simulink model "Simulink_PID_controller"  (R2024b)
settings: Solver=FixedStepDiscrete  StartTime=0.0  StopTime=Inf  FixedStep=1e-3  RelTol=1e-3  EnableMultiTasking=on
undefined symbols (not defined in the file): DiscIntNeverNeededParam
libraries: arduinolib x6, simulink x4, arduinosensorlib x2
settings Model: SimulationMode=external  ExtModeTrigDuration=2  Creator=Necus  LastModifiedBy=Rashmika Gunasekera
settings SolverCC: AutoInsertRateTranBlk=on
settings OptimizationCC: DefaultUnderspecifiedDataType=single  EnhancedBackFolding=on  PassReuseOutputArgsAs=Individual arguments  ZeroExternalMemoryAtStartup=off  MaxStackSize=64  OptimizeBlockOrder=speed  DifferentSizesBufferReuse=on  OptimizationCustomize=off  DenormalBehavior=FlushToZero  EfficientTunableParamExpr=on
settings DebuggingCC: ParameterTunabilityLossMsg=error
settings HardwareCC: ProdBitPerInt=16  ProdBitPerPointer=16  ProdBitPerSizeT=16  ProdBitPerPtrDiffT=16  ProdLargestAtomicFloat=None  ProdWordSize=8  ProdHWDeviceType=Atmel->AVR  UseEmbeddedCoderFeatures=off  UseSimulinkCoderFeatures=off
settings SFSimCC: MATLABDynamicMemAlloc=off
settings RTWCC: Description=Embedded Coder  SystemTargetFile=ert.tlc  HardwareBoard=Arduino Mega 2560  TemplateMakefile=ert_default_tmf  Toolchain=Arduino AVR  BuildConfiguration=Faster Runs  GPUComputeCapability=3.5
settings CodeAppCC: ForceParamTrailComments=on  IgnoreCustomStorageClasses=off  OperatorAnnotations=on  SimulinkDataObjDesc=on  SFDataObjDesc=on  InsertBlockDesc=on
settings ERTTargetCC: SupportContinuousTime=on  SupportNonInlinedSFcns=on  SupportVariableSizeSignals=on  ExtMode=on  ExtModeTransport=3  ExtModeStaticAlloc=on  ExtModeAutomaticAllocSize=off  ExtModeStaticAllocSize=2048  ExtModeMexFile=ext_xcp  ExtModeMexArgs=1 8 5625000  ExtModeIntrfLevel=Level2 - Open  InlinedParameterPlacement=Hierarchical  DynamicArrayContainerType=coder::array

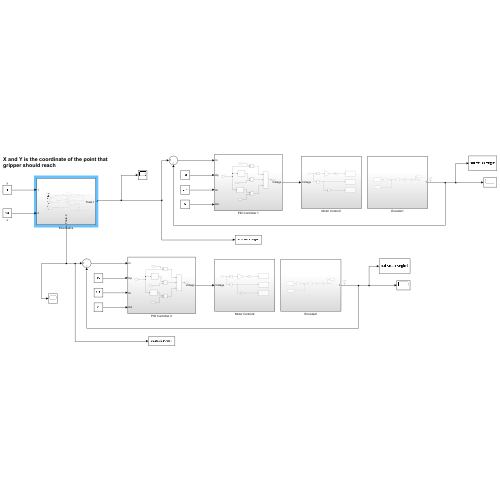
[thumbnail: Simulink's stored preview of the top-level diagram]
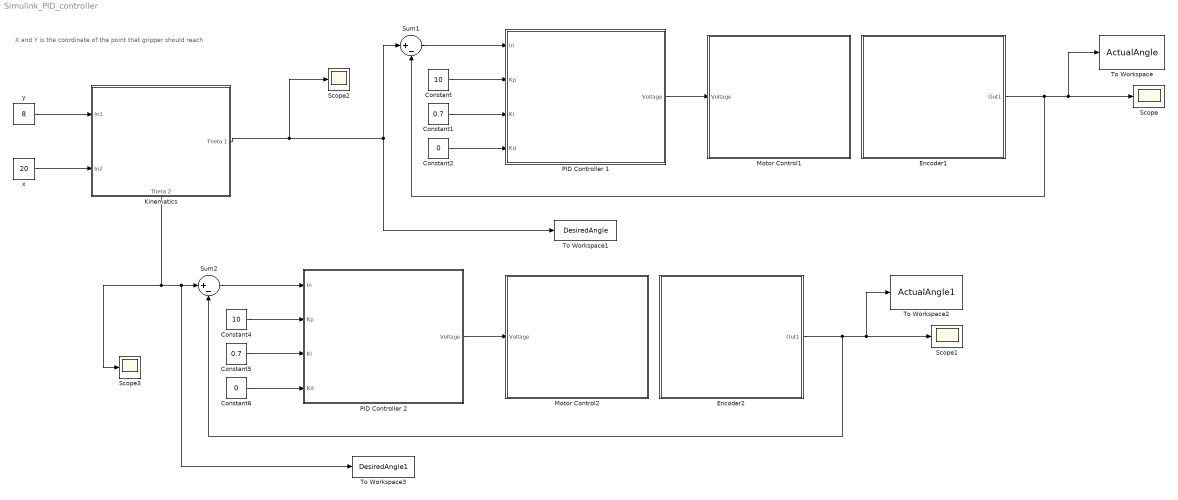
== system Simulink_PID_controller ==
  note: X and Y is the coordinate of the point that gripper should reach
  Constant : Constant  Value=10
  Constant1 : Constant  Value=0.7
  Constant2 : Constant  Value=0
  Constant4 : Constant  Value=10
  Constant5 : Constant  Value=0.7
  Constant6 : Constant  Value=0
  Encoder1 : Subsystem
  Encoder2 : Subsystem
  Kinematics : Subsystem
      settings: PortSchema="{\"entries\":[{\"content\":{\"sides\":[{\"content\":{\"connectorIds\":[\"In1\",\"In2\"]},\"type\":\"ConnectorPlacement.EquallySpacedRectSide\",\"uuid\":\"8a509842-5d2f-4ce8-a55f-cf93434b5f6d\"},{\"content\":{\"connectorIds\":[\"Out1\"],\"side\":\"RIGHT\"},\"type\":\"ConnectorPlacement.EquallySpacedRectSide\",\"uuid\":\"dc9cea0c-3903-48e2-b604-c30f542df696\"},{\"content\":{\"side\":\"TOP\"},\"type\":\"ConnectorPlacement.EquallySpacedRectSide\",\"uuid\":\"6c8ffbb7-f81a-45ff-8455-eba80b841fc4\"},{\"content\":{\"connectorIds\":[\"Out2\"],\"side\":\"BOTTOM\"},\"type\":\"ConnectorPlacement.EquallySpacedRectSide\",\"uuid\":\"0c610225-6bbf-4f4a-ad72-7adf458fb5c5\"}]},\"type\":\"ConnectorPlacement.EquallySpacedConnector\",\"uuid\":\"63fe37e8-0e78-4a01-8657-6f2a85bff4db\"}],\"packageUris\":[\"http://schema.mathworks.com/mf0/Connector/R2020b\"],\"version\":\"1.0\"}"
  Motor Control1 : Subsystem
  Motor Control2 : Subsystem
  PID Controller 1 : Subsystem
  PID Controller 2 : Subsystem
  Scope{,1..3} (4 alike) : Scope
  Sum1 : Sum  Inputs=|+-
  Sum2 : Sum  Inputs=|+-
  To Workspace : ToWorkspace  VariableName=ActualAngle  SaveFormat=Structure With Time  SampleTime=-1
  To Workspace1 : ToWorkspace  VariableName=DesiredAngle  SaveFormat=Structure With Time  SampleTime=-1
  To Workspace2 : ToWorkspace  VariableName=ActualAngle1  SaveFormat=Structure With Time  SampleTime=-1
  To Workspace3 : ToWorkspace  VariableName=DesiredAngle1  SaveFormat=Structure With Time  SampleTime=-1
  x : Constant  Value=20
  y : Constant  Value=8
  wires:
  Constant/1 -> PID Controller 1/2(Kp)
  Constant1/1 -> PID Controller 1/3(Ki)
  Constant2/1 -> PID Controller 1/4(Kd)
  Sum1/1 -> PID Controller 1/1(In)
  Encoder1/1(Out1) -> To Workspace/1, Scope/1, Sum1/2
  PID Controller 1/1(Voltage) -> Motor Control1/1(Voltage)
  Kinematics/2(Theta 2) -> To Workspace3/1, Sum2/1, Scope3/1
  Encoder2/1(Out1) -> To Workspace2/1, Scope1/1, Sum2/2
  Sum2/1 -> PID Controller 2/1(In)
  Constant6/1 -> PID Controller 2/4(Kd)
  Constant4/1 -> PID Controller 2/2(Kp)
  Constant5/1 -> PID Controller 2/3(Ki)
  PID Controller 2/1(Voltage) -> Motor Control2/1(Voltage)
  Kinematics/1(Theta 1) -> Scope2/1, To Workspace1/1, Sum1/1
  y/1 -> Kinematics/1(In1)
  x/1 -> Kinematics/2(In2)

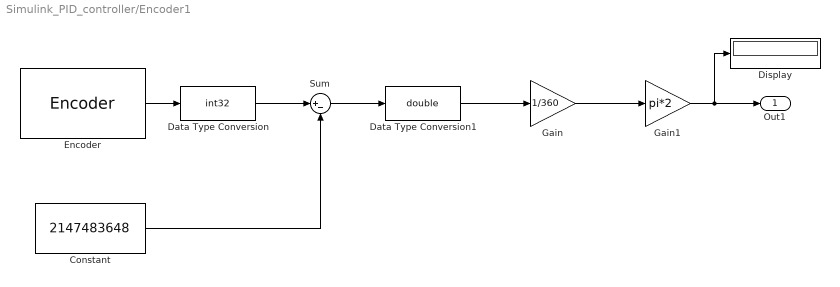
== system Simulink_PID_controller/Encoder1 ==
  Constant : Constant  Value=2147483648  OutDataTypeStr=int32
  Data Type Conversion : DataTypeConversion  OutDataTypeStr=int32  SaturateOnIntegerOverflow=off  RndMeth=Floor
  Data Type Conversion1 : DataTypeConversion  OutDataTypeStr=double  SaturateOnIntegerOverflow=off  RndMeth=Floor
  Display : Display
  Encoder : arduinosensorlib/Encoder  InputA=2  InputB=3  Mode=No reset  SampleTime=-1
      settings: SourceProductName=Sensors
  Gain : Gain  Gain=1/360
  Gain1 : Gain  Gain=pi*2
  Sum : Sum  Inputs=|+-
  Out1 : Outport
  wires:
  Data Type Conversion1/1 -> Gain/1
  Encoder/1 -> Data Type Conversion/1
  Data Type Conversion/1 -> Sum/1
  Sum/1 -> Data Type Conversion1/1
  Constant/1 -> Sum/2
  Gain/1 -> Gain1/1
  Gain1/1 -> Display/1, Out1/1

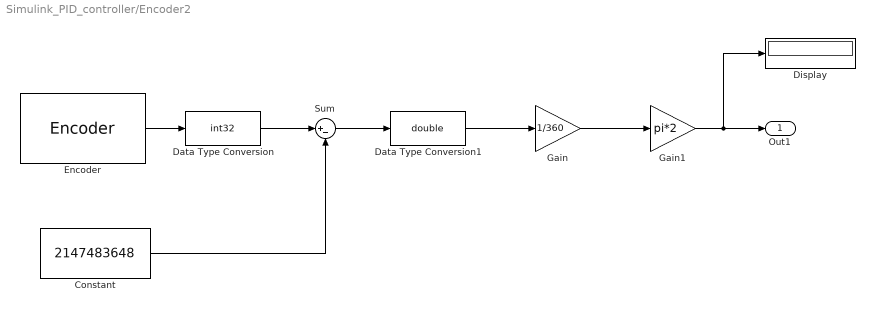
== system Simulink_PID_controller/Encoder2 ==
  Constant : Constant  Value=2147483648  OutDataTypeStr=int32
  Data Type Conversion : DataTypeConversion  OutDataTypeStr=int32  SaturateOnIntegerOverflow=off  RndMeth=Floor
  Data Type Conversion1 : DataTypeConversion  OutDataTypeStr=double  SaturateOnIntegerOverflow=off  RndMeth=Floor
  Display : Display
  Encoder : arduinosensorlib/Encoder  InputA=18  InputB=19  Mode=No reset  SampleTime=-1
      settings: SourceProductName=Sensors
  Gain : Gain  Gain=1/360
  Gain1 : Gain  Gain=pi*2
  Sum : Sum  Inputs=|+-
  Out1 : Outport
  wires:
  Data Type Conversion1/1 -> Gain/1
  Encoder/1 -> Data Type Conversion/1
  Data Type Conversion/1 -> Sum/1
  Sum/1 -> Data Type Conversion1/1
  Constant/1 -> Sum/2
  Gain/1 -> Gain1/1
  Gain1/1 -> Display/1, Out1/1

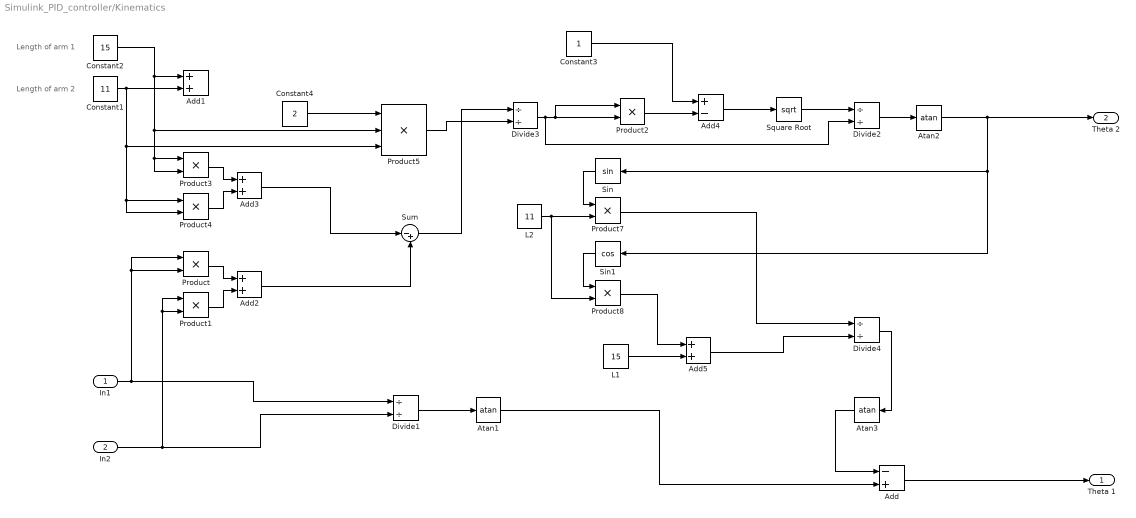
== system Simulink_PID_controller/Kinematics ==
  note: Length of arm 1
  note: Length of arm 2
  In1 : Inport
  In2 : Inport  Port=2
  Add : Sum  Inputs=-+
  Add{1..3,5} (4 alike) : Sum
  Add4 : Sum  Inputs=+-
  Atan1 : Trigonometry  Operator=atan
  Atan2 : Trigonometry  Operator=atan
  Atan3 : Trigonometry  Operator=atan
  Constant1 : Constant  Value=11
  Constant2 : Constant  Value=15
  Constant3 : Constant
  Constant4 : Constant  Value=2
  Divide{1..4} (4 alike) : Product  Inputs=//
  L1 : Constant  Value=15
  L2 : Constant  Value=11
  Product{,1..4,7..8} (7 alike) : Product
  Product5 : Product  Inputs=3
  Sin : Trigonometry
  Sin1 : Trigonometry  Operator=cos
  Square Root : Sqrt
  Sum : Sum  Inputs=|-+
  Theta 1 : Outport
  Theta 2 : Outport  Port=2
  wires:
  In2/1 -> Divide1/2, Product1/2, Product1/1
  In1/1 -> Product/2, Product/1, Divide1/1
  Divide1/1 -> Atan1/1
  Add/1 -> Theta 1/1
  Constant2/1 -> Product3/1, Product3/2, Product5/2, Add1/1
  Constant1/1 -> Product4/1, Product4/2, Product5/3, Add1/2
  Product/1 -> Add2/1
  Product1/1 -> Add2/2
  Product4/1 -> Add3/2
  Product3/1 -> Add3/1
  Add2/1 -> Sum/2
  Add3/1 -> Sum/1
  Sum/1 -> Divide3/1
  Constant4/1 -> Product5/1
  Product5/1 -> Divide3/2
  Atan1/1 -> Add/2
  Divide3/1 -> Product2/2, Product2/1, Divide2/2
  Product2/1 -> Add4/2
  Constant3/1 -> Add4/1
  Add4/1 -> Square Root/1
  Square Root/1 -> Divide2/1
  Divide2/1 -> Atan2/1
  Atan2/1 -> Theta 2/1, Sin1/1, Sin/1
  L2/1 -> Product8/2, Product7/2
  Sin/1 -> Product7/1
  Sin1/1 -> Product8/1
  L1/1 -> Add5/2
  Product8/1 -> Add5/1
  Product7/1 -> Divide4/1
  Add5/1 -> Divide4/2
  Divide4/1 -> Atan3/1
  Atan3/1 -> Add/1

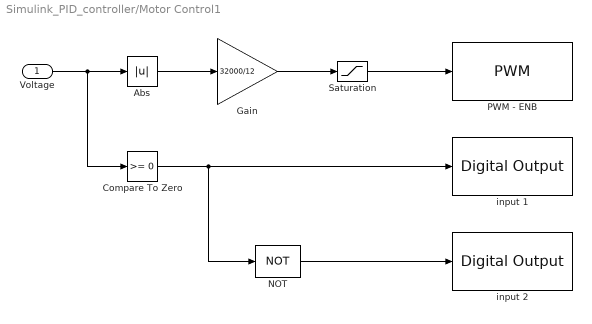
== system Simulink_PID_controller/Motor Control1 ==
  Voltage : Inport
  Abs : Abs  SaturateOnIntegerOverflow=off
  Compare To Zero : simulink/Logic and Bit Operations/Compare To Zero  relop=>=  OutDataTypeStr=boolean
  Gain : Gain  Gain=32000/12
  NOT : Logic  Operator=NOT  IconShape=distinctive  AllPortsSameDT=off  OutDataTypeStr=boolean
  PWM - ENB : arduinolib/PWM  pinNumber=7  frequencyType=Default  desiredFrequency=490.2  achievableFrequency=490.2
      settings: SourceProductName=Common
  Saturation : Saturate  UpperLimit=32000  LowerLimit=0
  "input 1 " : arduinolib/Digital Output  pinNumber=5  Direction=output  blockPlatform=arduino
      settings: SourceProductName=Common
  input 2 : arduinolib/Digital Output  pinNumber=6  Direction=output  blockPlatform=arduino
      settings: SourceProductName=Common
  wires:
  Voltage/1 -> Compare To Zero/1, Abs/1
  Abs/1 -> Gain/1
  Gain/1 -> Saturation/1
  Compare To Zero/1 -> "input 1 "/1, NOT/1
  NOT/1 -> input 2/1
  Saturation/1 -> PWM - ENB/1

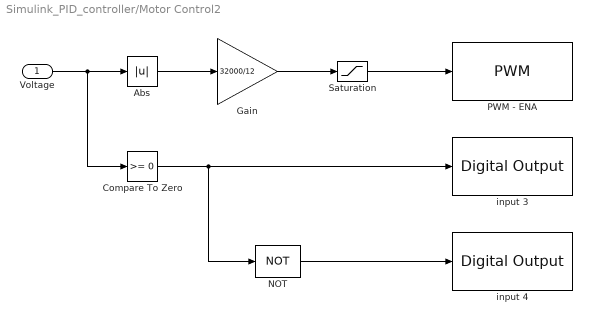
== system Simulink_PID_controller/Motor Control2 ==
  Voltage : Inport
  Abs : Abs  SaturateOnIntegerOverflow=off
  Compare To Zero : simulink/Logic and Bit Operations/Compare To Zero  relop=>=  OutDataTypeStr=boolean
  Gain : Gain  Gain=32000/12
  NOT : Logic  Operator=NOT  IconShape=distinctive  AllPortsSameDT=off  OutDataTypeStr=boolean
  PWM - ENA : arduinolib/PWM  pinNumber=8  frequencyType=Default  desiredFrequency=490.2  achievableFrequency=490.2
      settings: SourceProductName=Common
  Saturation : Saturate  UpperLimit=32000  LowerLimit=0
  "input 3 " : arduinolib/Digital Output  pinNumber=9  Direction=output  blockPlatform=arduino
      settings: SourceProductName=Common
  input 4 : arduinolib/Digital Output  pinNumber=10  Direction=output  blockPlatform=arduino
      settings: SourceProductName=Common
  wires:
  Voltage/1 -> Compare To Zero/1, Abs/1
  Abs/1 -> Gain/1
  Gain/1 -> Saturation/1
  Compare To Zero/1 -> "input 3 "/1, NOT/1
  NOT/1 -> input 4/1
  Saturation/1 -> PWM - ENA/1

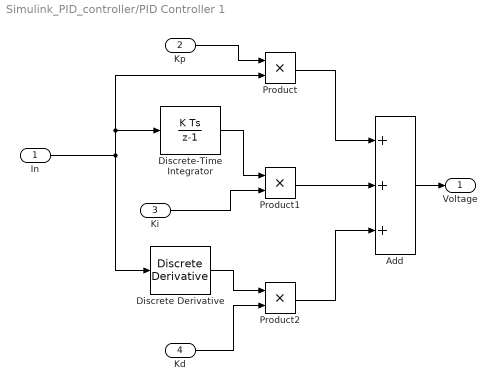
== system Simulink_PID_controller/PID Controller 1 ==
  In : Inport
  Kp : Inport  Port=2
  Ki : Inport  Port=3
  Kd : Inport  Port=4
  Add : Sum  Inputs=+++
  Discrete Derivative : simulink/Discrete/Discrete Derivative  gainval=1.0  ICPrevScaledInput=0.0  OutMin=[]  OutMax=[]  OutDataType=fixdt(1, 16)  OutScaling=2^-10  DoSatur=off
  Discrete-Time Integrator : DiscreteIntegrator  SampleTime=-1  ICPrevOutput=DiscIntNeverNeededParam  ICPrevScaledInput=DiscIntNeverNeededParam
  Product : Product
  Product1 : Product
  Product2 : Product
  Voltage : Outport
  wires:
  Discrete-Time Integrator/1 -> Product1/1
  Product2/1 -> Add/3
  Ki/1 -> Product1/2
  Discrete Derivative/1 -> Product2/1
  In/1 -> Product/2, Discrete-Time Integrator/1, Discrete Derivative/1
  Kd/1 -> Product2/2
  Product/1 -> Add/1
  Product1/1 -> Add/2
  Kp/1 -> Product/1
  Add/1 -> Voltage/1

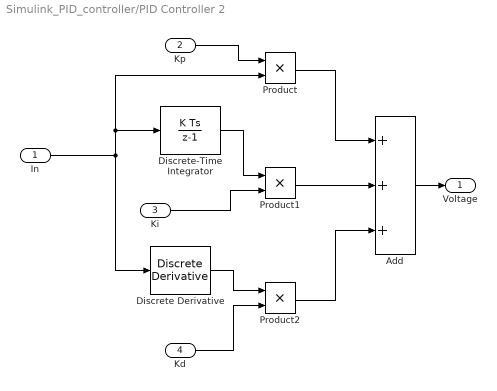
== system Simulink_PID_controller/PID Controller 2 ==
  In : Inport
  Kp : Inport  Port=2
  Ki : Inport  Port=3
  Kd : Inport  Port=4
  Add : Sum  Inputs=+++
  Discrete Derivative : simulink/Discrete/Discrete Derivative  gainval=1.0  ICPrevScaledInput=0.0  OutMin=[]  OutMax=[]  OutDataType=fixdt(1, 16)  OutScaling=2^-10  DoSatur=off
  Discrete-Time Integrator : DiscreteIntegrator  SampleTime=-1  ICPrevOutput=DiscIntNeverNeededParam  ICPrevScaledInput=DiscIntNeverNeededParam
  Product : Product
  Product1 : Product
  Product2 : Product
  Voltage : Outport
  wires:
  Discrete-Time Integrator/1 -> Product1/1
  Product2/1 -> Add/3
  Ki/1 -> Product1/2
  Discrete Derivative/1 -> Product2/1
  In/1 -> Product/2, Discrete-Time Integrator/1, Discrete Derivative/1
  Kd/1 -> Product2/2
  Product/1 -> Add/1
  Product1/1 -> Add/2
  Kp/1 -> Product/1
  Add/1 -> Voltage/1
